simulink model "LQ_model"  (R2017b)
settings: Solver=ode45  StartTime=0.0  StopTime=50  RelTol=1e-3  EnableMultiTasking=on
values from neighbouring files (symbols this model uses):
  angle1 = 0    [LQ_main.m]
  angle2 = 0    [LQ_main.m]
  h = 0.001    [LQ_main.m]
  K = K_lqi(1:4)    [LQ_main.m]
  Ki = K_lqi(5:6)    [LQ_main.m]
  Q_kal = 10^(-9)*[100 1 1 1; 1 100 1 1; 1 1 100 1; 1 1 1 100]    [LQ_main.m]
  R_kal = cov(err)    [LQ_main.m]
undefined symbols (not defined in the file or in its folder): adingain, adinoffs, daoutgain, daoutoffs, DiscIntNeverNeededParam, Discrete, Time
libraries: ctrlSharedLib x1
settings Model: Creator=rbabuska  LastModifiedBy=Stein
settings DataIOCC: LimitDataPoints=on  SaveFormat=Array  SignalLoggingName=sigsOut
settings OptimizationCC: BooleanDataType=off  ExpressionDepthLimit=2147483647  InitFltsAndDblsToZero=on  LifeSpan=inf
settings DebuggingCC: SaveWithParameterizedLinksMsg=none  SignalResolutionControl=TryResolveAllWithWarning  MultiTaskDSMMsg=warning  MultiTaskCondExecSysMsg=none  AllowSymbolicDim=off  StateNameClashWarn=warning  SFUnexpectedBacktrackingDiag=warning  SFNoUnconditionalDefaultTransitionDiag=warning  SFExecutionAtInitializationDiag=none
settings HardwareCC: ProdBitPerPointer=32  ProdBitPerSizeT=32  ProdBitPerPtrDiffT=32  ProdLargestAtomicFloat=None  ProdIntDivRoundTo=Undefined  ProdEndianess=Unspecified  ProdWordSize=32  ProdHWDeviceType=32-bit Generic  TargetUnknown=on
settings ModelReferenceCC: PropagateSignalLabelsOutOfModel=off
settings CodeAppCC: StateflowObjectComments=on
settings GRTTargetCC: TargetFcnLib=ansi_tfl_tmw.mat  TargetLangStandard=C89/C90 (ANSI)  GeneratePreprocessorConditionals=Disable all  CombineOutputUpdateFcns=off  GRTInterface=on
settings ConfigComp: CovMetricSettings=dw  CovHtmlReporting=on  CovSaveCumulativeToWorkspaceVar=on  CovSaveSingleToWorkspaceVar=on  CovExternalEMLEnable=off

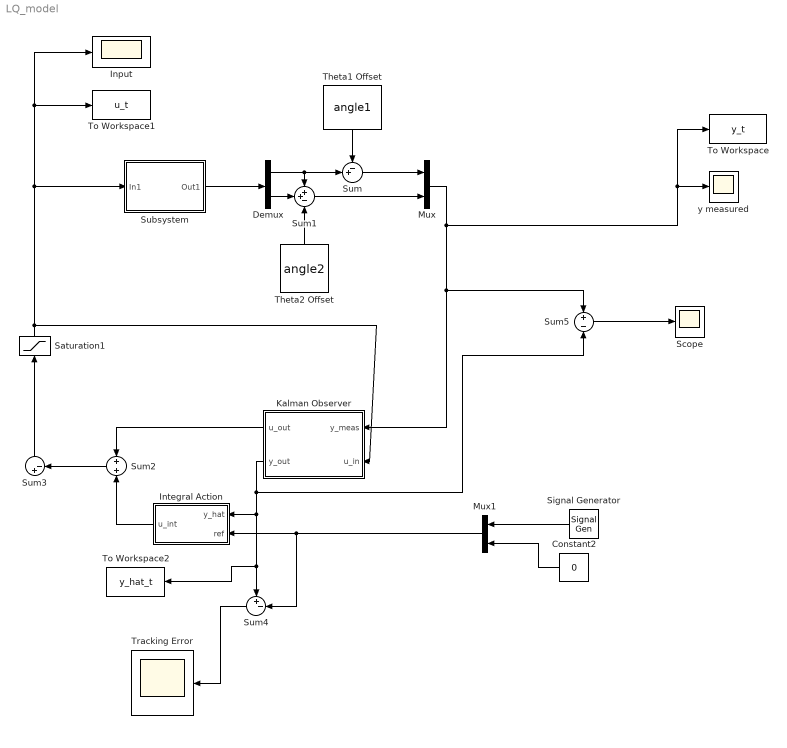
== system LQ_model ==
  Constant2 : Constant  Value=0
  Demux : Demux  Outputs=2
  Input : Scope
  Integral Action : Subsystem
  Kalman Observer : Subsystem
  Mux : Mux  Inputs=2
  Mux1 : Mux  Inputs=2
  Saturation1 : Saturate  UpperLimit=1  LowerLimit=-1
  Scope : Scope
  Signal Generator : SignalGenerator  Amplitude=0.5  Frequency=0.6  Units=rad/sec
  Subsystem : Subsystem
      mask Display: disp('Rotational\nPendulum')
  Sum : Sum  Inputs=-+|
  Sum1 : Sum  Inputs=++-
  Sum2 : Sum
  Sum3 : Sum  Inputs=|+-
  Sum4 : Sum  Inputs=+-|
  Sum5 : Sum  Inputs=+-
  Theta1 Offset : Constant  Value=angle1
  Theta2 Offset : Constant  Value=angle2
  To Workspace : ToWorkspace  VariableName=y_t  SaveFormat=Timeseries  SampleTime=-1
  To Workspace1 : ToWorkspace  VariableName=u_t  SaveFormat=Timeseries  SampleTime=-1
  To Workspace2 : ToWorkspace  VariableName=y_hat_t  SaveFormat=Timeseries  SampleTime=-1
  Tracking Error : Scope
  y measured : Scope
  wires:
  Demux/1 -> Sum/2, Sum1/1
  Mux/1 -> Kalman Observer/1(y_meas), Sum5/1, To Workspace/1, y measured/1
  Subsystem/1(Out1) -> Demux/1
  Theta1 Offset/1 -> Sum/1
  Sum/1 -> Mux/1
  Kalman Observer/1(u_out) -> Sum2/1
  Kalman Observer/2(y_out) -> Integral Action/1(y_hat), To Workspace2/1, Sum4/1, Sum5/2
  Integral Action/1(u_int) -> Sum2/2
  Sum2/1 -> Sum3/2
  Constant2/1 -> Mux1/2
  Mux1/1 -> Integral Action/2(ref), Sum4/2
  Sum4/1 -> Tracking Error/1
  Demux/2 -> Sum1/2
  Theta2 Offset/1 -> Sum1/3
  Sum5/1 -> Scope/1
  Saturation1/1 -> Kalman Observer/2(u_in), Input/1, To Workspace1/1, Subsystem/1(In1)
  Sum1/1 -> Mux/2
  Sum3/1 -> Saturation1/1
  Signal Generator/1 -> Mux1/1

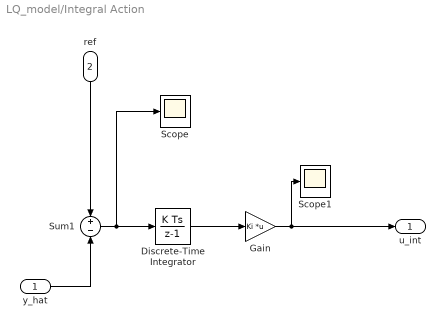
== system LQ_model/Integral Action ==
  y_hat : Inport
  ref : Inport  Port=2
  Discrete-Time Integrator : DiscreteIntegrator  gainval=1  InitialConditionSetting=State (most efficient)  SampleTime=h  ICPrevOutput=DiscIntNeverNeededParam  ICPrevScaledInput=DiscIntNeverNeededParam
  Gain : Gain  Gain=Ki  Multiplication=Matrix(K*u)
  Scope : Scope
  Scope1 : Scope
  Sum1 : Sum  Inputs=+-
  u_int : Outport
  wires:
  ref/1 -> Sum1/1
  y_hat/1 -> Sum1/2
  Sum1/1 -> Scope/1, Discrete-Time Integrator/1
  Discrete-Time Integrator/1 -> Gain/1
  Gain/1 -> Scope1/1, u_int/1

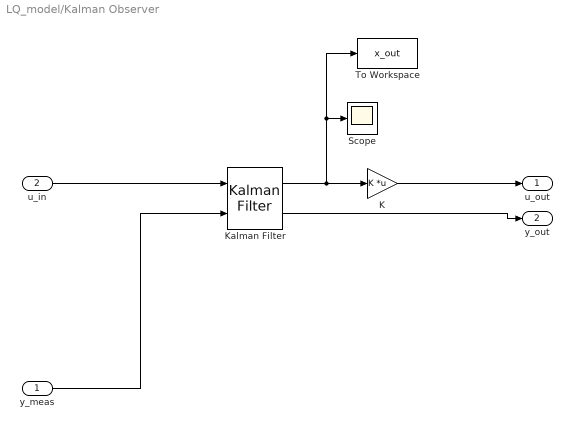
== system LQ_model/Kalman Observer ==
  y_meas : Inport
  u_in : Inport  Port=2
  K : Gain  Gain=K  Multiplication=Matrix(K*u)
  Kalman Filter : ctrlSharedLib/Kalman Filter  TimeDomain=Discrete-Time  UseCurrentEstimator=on  ModelSource=LTI State-Space Variable  ModelSourceVariable=sysd  A=0.95  B=1  C=1  D=0  NumberOfStates=1  NumberOfInputs=1  NumberOfOutputs=1  InitialEstimateSource=Dialog  X0=[0 0 0 0]  P0=10  UseK=off  UseGH=off  NumberOfProcessNoiseInputs=1  G=1  TimeInvariantG=on  H=0  TimeInvariantH=on  Q=Q_kal/1000  TimeInvariantQ=on  R=R_kal  TimeInvariantR=on  N=0  TimeInvariantN=on  AddInputPort=on  AddEnablePort=off  OutputEstimatedY=on  OutputP=off  Ts=-1
      settings: SourceProductBaseCode=CT
  Scope : Scope
  To Workspace : ToWorkspace  VariableName=x_out  SaveFormat=Timeseries  SampleTime=-1
  u_out : Outport
  y_out : Outport  Port=2
  wires:
  K/1 -> u_out/1
  u_in/1 -> Kalman Filter/1
  Kalman Filter/2 -> y_out/1
  y_meas/1 -> Kalman Filter/2
  Kalman Filter/1 -> To Workspace/1, Scope/1, K/1

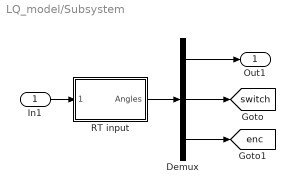
== system LQ_model/Subsystem ==
  In1 : Inport
  Demux : Demux  Outputs=[2 4 1]
  RT input : Subsystem  mask{Ts=h, channels=[6 7]}
      mask prompts: Ts "Sample time [s]:"; channels "Channels to read (e.g., [6 7])"
      mask init:
      | hwinit;
      | 
      | % initialize FPGA
      | fugihandle = fugiboard('Open', 'Pendulum1');
      | fugihandle.WatchdogTimeout = 0.5;
      | fugiboard('SetParams', fugihandle);
      | fugiboard('Write', fugihandle, 0, 0, 0, 0);  % dummy write to sync interface board
      | fugiboard('Write', fugihandle, 5, 1, 0, 0);  % reset position, activate relay
      | data = fugiboard('Read', fugihandle);        % get version info from FPGA
      | % model = bitshift(data(1), -5); 
      | % version = bitand(data(1), 31);
      | % disp(sprintf('FPGA setup %d, version %d', model, version)); % for the B&P it should say 1 1, or else there is a problem
      | fugiboard('Write', fugihandle, 0, 1, 0, 0);  % end reset
      | pause(0.1);                         % give relay some time to respond
      mask Display: disp('Rotational\nPendulum')
  Out1 : Outport
  tag scope: enc=global, switch=global
  wires:
  RT input/1(Angles) -> Demux/1
  Demux/1 -> Out1/1
  Demux/2 -> [switch]
  Demux/3 -> [enc]
  In1/1 -> RT input/1(Motors)

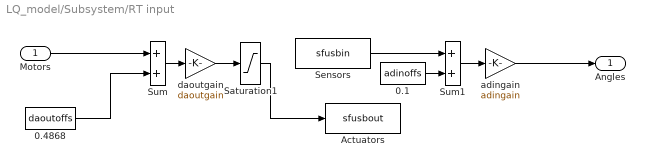
== system LQ_model/Subsystem/RT input ==
  Motors : Inport
  0.1 : Constant  Value=adinoffs
  0.4868 : Constant  Value=daoutoffs
  Actuators : S-Function  FunctionName=sfusbout  Parameters=Ts, fugihandle  SFunctionDeploymentMode=off  EnableBusSupport=off
  Saturation1 : Saturate  UpperLimit=10  LowerLimit=-10
  Sensors : S-Function  FunctionName=sfusbin  Parameters=Ts, fugihandle, channels  SFunctionDeploymentMode=off  EnableBusSupport=off
  Sum : Sum  SaturateOnIntegerOverflow=on  InputSameDT=on  OutDataTypeStr=Inherit: Same as first input
  Sum1 : Sum  SaturateOnIntegerOverflow=on  InputSameDT=on  OutDataTypeStr=Inherit: Same as first input
  adingain : Gain  Gain=adingain  SaturateOnIntegerOverflow=on  OutDataTypeStr=Inherit: Same as input  ParamDataTypeStr=Inherit: Same as input
  daoutgain : Gain  Gain=daoutgain  SaturateOnIntegerOverflow=on  OutDataTypeStr=Inherit: Same as input  ParamDataTypeStr=Inherit: Same as input
  Angles : Outport
  wires:
  Sum/1 -> daoutgain/1
  0.4868/1 -> Sum/2
  Motors/1 -> Sum/1
  Sum1/1 -> adingain/1
  0.1/1 -> Sum1/2
  Sensors/1 -> Sum1/1
  adingain/1 -> Angles/1
  Saturation1/1 -> Actuators/1
  daoutgain/1 -> Saturation1/1
